simulink model "P7simulink"  (R2024b)
settings: Solver=VariableStepAuto  StartTime=0.0  StopTime=10  RelTol=1e-3
InitFcn:
  | R1=5000000;
  | R2=5000000;
  | R3=5000000;
  | C1=.0000001;
  | C2=.0000001;
settings Model: Creator=Becho

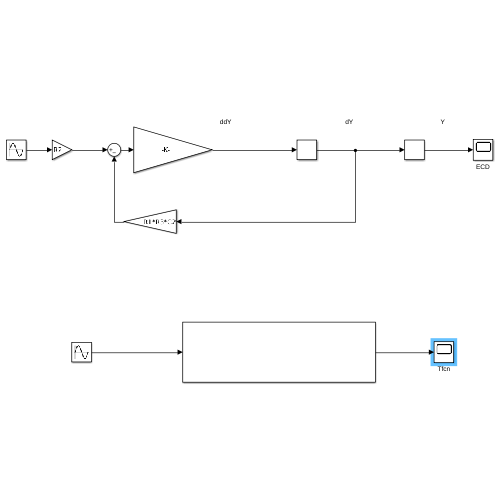
[thumbnail: Simulink's stored preview of the top-level diagram]
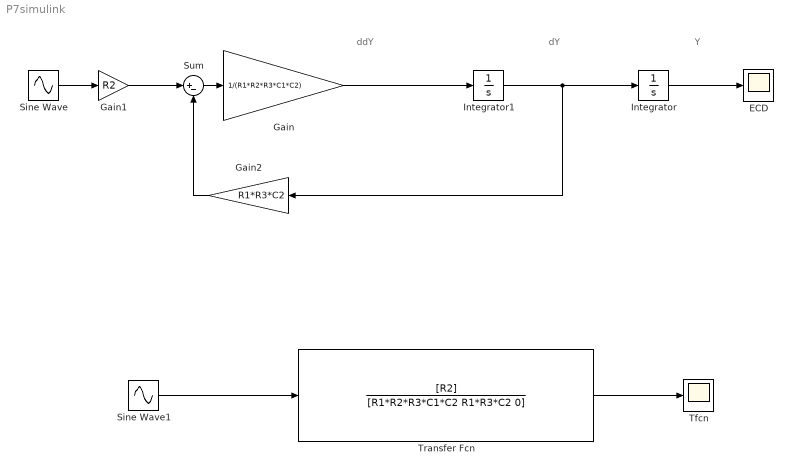
== system P7simulink ==
  note: ddY
  note: dY
  note: Y
  ECD : Scope
  Gain : Gain  Gain=1/(R1*R2*R3*C1*C2)
  Gain1 : Gain  Gain=R2
  Gain2 : Gain  Gain=R1*R3*C2
  Integrator : Integrator
  Integrator1 : Integrator
  Sine Wave : Sin  Frequency=628.318530718  SampleTime=0
  Sine Wave1 : Sin  Frequency=628.318530718  SampleTime=0
  Sum : Sum  Inputs=|+-
  Tfcn : Scope
  Transfer Fcn : TransferFcn  Numerator=[R2]  Denominator=[R1*R2*R3*C1*C2 R1*R3*C2 0]
  wires:
  Integrator1/1 -> Gain2/1, Integrator/1
  Gain/1 -> Integrator1/1
  Sum/1 -> Gain/1
  Sine Wave/1 -> Gain1/1
  Gain1/1 -> Sum/1
  Gain2/1 -> Sum/2
  Integrator/1 -> ECD/1
  Sine Wave1/1 -> Transfer Fcn/1
  Transfer Fcn/1 -> Tfcn/1
